simulink model "AariaHIABR2017a"  (R2017a)
settings: Solver=VariableStepAuto  StartTime=0.0  StopTime=inf  FixedStep=0.1  RelTol=1e-3  EnableMultiTasking=on
model workspace (MATLAB code in the model file):
  | my_a =1;
undefined symbols (not defined in the file or in its folder): AARIAENV, AARIAMAN, AARIASEN, Camera, sensor, Source_TS, X, Y, Z
libraries: sm_lib x347, nesl_utility x194, dspmathops x74, simulink x72, vrlib x2, powerlib_meascontrol x1, aerolibanimutils x1, aerolibutil x1
(part 1 of 9)
settings Model: Creator=mohmmadi  LastModifiedBy=hautakos
settings SolverCC: ZeroCrossControl=DisableAll  AutoInsertRateTranBlk=on
settings DataIOCC: LimitDataPoints=on  SaveOutput=off  SaveTime=off  ReturnWorkspaceOutputs=on
settings OptimizationCC: DefaultParameterBehavior=Inlined  InlineInvariantSignals=on  PassReuseOutputArgsThreshold=0  StateBitsets=on  DataBitsets=on  EfficientMapNaN2IntZero=off  LifeSpan=1
settings DebuggingCC: ReadBeforeWriteMsg=DisableAll  WriteAfterWriteMsg=DisableAll  WriteAfterReadMsg=DisableAll  MultiTaskDSMMsg=none  ParameterTunabilityLossMsg=error  AllowSymbolicDim=off  SFUnexpectedBacktrackingDiag=warning  SFNoUnconditionalDefaultTransitionDiag=warning  SFExecutionAtInitializationDiag=none
settings HardwareCC: ProdBitPerPointer=32  ProdBitPerSizeT=32  ProdBitPerPtrDiffT=32  ProdLargestAtomicFloat=None  ProdIntDivRoundTo=Floor  ProdWordSize=32  ProdHWDeviceType=Generic->Custom  TargetBitPerPointer=64  TargetBitPerSizeT=64  TargetBitPerPtrDiffT=64  TargetLongLongMode=on  TargetIntDivRoundTo=Zero  TargetEndianess=LittleEndian  TargetWordSize=64  TargetHWDeviceType=MATLAB Host  ProdEqTarget=off
settings ModelReferenceCC: UpdateModelReferenceTargets=IfOutOfDate  PropagateSignalLabelsOutOfModel=off
settings SFSimCC: SFSimEcho=off  MATLABDynamicMemAlloc=off
settings CodeAppCC: MaxIdLength=128
settings GRTTargetCC: TargetLangStandard=C89/C90 (ANSI)  CombineOutputUpdateFcns=off  GRTInterface=on
settings ConfigComp: CovMetricSettings=dw  CovHtmlReporting=on  CovSaveCumulativeToWorkspaceVar=on  CovSaveSingleToWorkspaceVar=on  CovExternalEMLEnable=off
settings ConfigurationSet: Description=SimMechanics 2G
settings ExplorerConfigSet: InternalSimMechanicsExplorerSettings="<ExplorerConfiguration><canonicalview>default</canonicalview><AnimationSetting><BasePlaybackSpeed>1.0</BasePlaybackSpeed><PlaybackSpeedFactor>2.0</PlaybackSpeedFactor></AnimationSetting><TilePanel><TileInfo><Tiles Columns=\"1\" Count=\"2\" Rows=\"2\"><Column Left=\"2\" Weight=\"1\"/><Column Left=\"662\"/><Row Top=\"2\" Weight=\"0.0567\"/><Row Top=\"65\" Weight=\"0.9433\"/><Row Top=\"1044\"/><Tile Height=\"1\" Width=\"1\" X=\"0\" Y=\"0\"/><Tile Height=\"1\" Width=\"1\" X=\"0\" Y=\"1\"/></Tiles></TileInfo><SceneInfo><SceneViewer><BGColor><R>0.60000002384185791</R><G>0.60000002384185791</G><B>0.60000002384185791</B></BGColor><Camera><DoPerspective>on</DoPerspective><Position><X>0.29999999999996857</X><Y>0.67968092512139899</Y><Z>1.3121696311764592</Z></Position><Center><X>-0.40710678118653471</X><Y>0.96126383425833517</Y><Z>1.9607920677927408</Z></Center><Up><X>-0.70710678118659176</X><Y>-0.28158290913685957</Y><Z>-0.64862243661621855</Z></Up><ViewLimDist>1</ViewLimDist><YLim>0.46630765815499858</YLim><XLim>5.6215978788685943</XLim></Camera></SceneViewer><SceneViewer><BGColor><R>0.60000002384185791</R><G>0.60000002384185791</G><B>0.60000002384185791</B></BGColor><Camera><DoPerspective>off</DoPerspective><Position><X>11.797763851673334</X><Y>-2.3957368450041248</Y><Z>7.7621866671693311</Z></Position><Center><X>-0.83316578837101418</X><Y>0.55050667633401429</Y><Z>1.2511357928731988</Z></Center><Up><X>-0.41467681338169138</X><Y>0.18924346197555764</Y><Z>0.89007306022770494</Z></Up><ViewLimDist>1</ViewLimDist><YLim>3.9492259066518822</YLim><XLim>2.6504598610622425</XLim></Camera></SceneViewer></SceneInfo></TilePanel><MechEditorPanel><Cameras><Camera><Id>Camera1</Id><Value><Name>Camera1</Name><NativeCamera><PositionTrackingFeature>Tool.Camera.R</PositionTrackingFeature><CenterTrackingFeature>Tool.Camera.R</CenterTrackingFeature><UpVectorTrackingFeature>Tool.Camera.R</UpVectorTrackingFeature><CenterTrackingOrigin>off</CenterTrackingOrigin><CenterTrackingDirection>+X</CenterTrackingDirection><UpVectorTrackingDirection>+Z</UpVectorTrackingDirection></NativeCamera></Value></Camera></Cameras><GfxPanelCameraMap><MapElement CameraMLId=\"Camera1\" GfxPanelIndex=\"0\"/></GfxPanelCameraMap><VideoCreator><PlaybackSpeedRatio>1.0</PlaybackSpeedRatio><FrameRate>30</FrameRate><VideoFormat>Motion JPEG AVI</VideoFormat><FrameSize>auto</FrameSize></VideoCreator></MechEditorPanel></ExplorerConfiguration>"

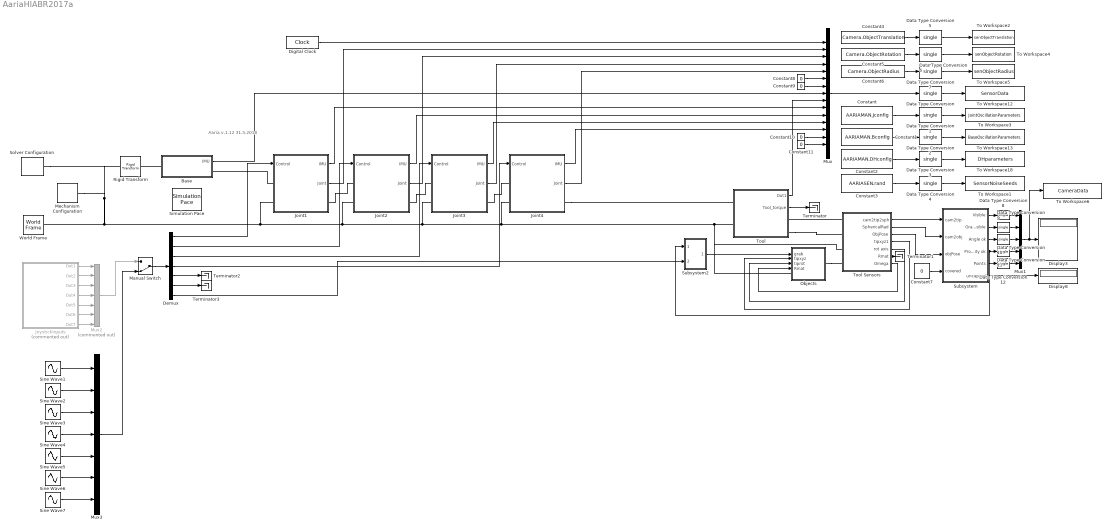
== system AariaHIABR2017a ==
  note: Aaria v.1.12
      | 31.5.2018
  Base : Subsystem  mask{Link_number=8}
  Constant : Constant  Value=AARIAMAN.Jconfig  VectorParams1D=off
  Constant1 : Constant  Value=AARIAMAN.Bconfig  VectorParams1D=off
  Constant{7..11} (5 alike) : Constant  Value=0
  Constant2 : Constant  Value=AARIAMAN.DHconfig  VectorParams1D=off  OutDataTypeStr=double
  Constant3 : Constant  Value=AARIASEN.rand  VectorParams1D=off  OutDataTypeStr=double
  Constant4 : Constant  Value=Camera.ObjectTranslation
  Constant5 : Constant  Value=Camera.ObjectRotation
  Constant6 : Constant  Value=Camera.ObjectRadius
  Data Type Conversion{,1..12} (13 alike) : DataTypeConversion  OutDataTypeStr=single
  Demux : Demux  Outputs=7
  Digital Clock : DigitalClock  SampleTime=AARIAENV.Sensor_TS
  Display3 : Display
  Display8 : Display
  Joint1 : Subsystem  mask{Link_number=1}
  Joint2 : Subsystem  mask{Link_number=2}
  Joint3 : Subsystem  mask{Link_number=3}
  Joint4 : Subsystem  mask{Link_number=4}
  JoystickInputs : Subsystem  Commented=on
  Manual Switch : ManualSwitch  CurrentSetting=0
  Mechanism Configuration : sm_lib/Utilities/Mechanism Configuration  UniformGravity=Constant  GravityVector=AARIAENV.gravity  GravityUnits=m/s^2  LinearizationDelta=0.001
  Mux : Mux  Inputs=15
  Mux1 : Mux  Inputs=5
  Mux2 : Mux  Commented=on  Inputs=7
  Mux3 : Mux  Inputs=7
  Objects : Subsystem
  Rigid Transform : sm_lib/Frames and Transforms/Rigid Transform  TranslationMethod=None  TranslationStandardOffset=0  TranslationLengthUnit=m  TranslationStandardAxis=+Z  TranslationCartesianOffset=[0 0 0.01]  TranslationROffset=0  TranslationROffsetUnits=m  TranslationZOffset=0  TranslationZOffsetUnits=m  TranslationThetaOffset=0  TranslationThetaOffsetUnits=deg  RotationMethod=StandardAxis  RotationAngleUnits=rad  RotationStandardAxis=+X  RotationAngle=-pi/2  RotationArbitraryAxis=[0 0 1]  FollAlignAxisA=+X  BaseAlignAxisA=+Y  FollAlignAxisB=+Y  BaseAlignAxisB=+Z  RotationSequenceAxes=FollowerAxes  RotationSequence=XYX  RotationSequenceAngles=[0 0 0]  RotationSequenceAnglesUnits=deg  RotationMatrix=[1 0 0; 0 1 0; 0 0 1]
  Simulation Pace : aerolibanimutils/Simulation Pace  SimulationPace=1  SleepMode=MATLAB Thread  OutputPaceError=off  SampleTime=1/30
  Sine Wave{1..7} (7 alike) : Sin  SampleTime=AARIAENV.Source_TS
  Solver Configuration : nesl_utility/Solver Configuration  PhysicalDomain=network_engine_domain  SubClassName=solver  LeftPortType=input  RightPortType=generic  Accelerate=off  Tones=[]  Harmonics=[]  SimulateNoise=off  Profile=off  UseLocalSampling=off  EnableSwitchedLinearOptims=on  FrequencyDomain=off  UseCCode=off  RelTol=0.001  AbsTol=1e-06  MinStep=1e-09  ToWorkspace=off  RevertToSquareIcSolve=off  NumHomotopyIterations=100  PhasorMode=off  PhasorModeNumHarmonics=1  OverrideAbsTol=off  DoDC=off  ResidualTolerance=1e-09  UseLocalSolver=off  LocalSolverChoice=NE_BACKWARD_EULER_ADVANCER  LocalSolverSampleTime=0.001  DoFixedCost=off  MaxNonlinIter=3  MaxModeIter=2  LinearAlgebra=Sparse  DelaysMemoryBudget=1024  AutomaticFiltering=on  FilteringTimeConstant=0.001
  Subsystem : Subsystem
  Subsystem2 : Subsystem
  Terminator{,1..3} (4 alike) : Terminator
  To Workspace1 : ToWorkspace  VariableName=SensorNoiseSeeds  SampleTime=AARIAENV.Sensor_TS
      settings: MaxDataPoints=8  Save2DSignal=2-D array (concatenate along first dimension)
  To Workspace12 : ToWorkspace  VariableName=SensorData  SampleTime=AARIAENV.Sensor_TS
      settings: Save2DSignal=2-D array (concatenate along first dimension)
  To Workspace13 : ToWorkspace  VariableName=BaseOscillationParameters  SampleTime=AARIAENV.Sensor_TS
      settings: MaxDataPoints=24  Save2DSignal=2-D array (concatenate along first dimension)
  To Workspace18 : ToWorkspace  VariableName=DHparameters  SampleTime=AARIAENV.Sensor_TS
      settings: MaxDataPoints=8  Save2DSignal=2-D array (concatenate along first dimension)
  To Workspace2 : ToWorkspace  VariableName=senObjectTranslation  SampleTime=AARIAENV.Sensor_TS
      settings: MaxDataPoints=1  Save2DSignal=2-D array (concatenate along first dimension)
  To Workspace3 : ToWorkspace  VariableName=JointOscillationParameters  SampleTime=AARIAENV.Sensor_TS
      settings: MaxDataPoints=6  Save2DSignal=2-D array (concatenate along first dimension)
  To Workspace4 : ToWorkspace  VariableName=senObjectRotation  SampleTime=AARIAENV.Sensor_TS
      settings: MaxDataPoints=3  Save2DSignal=2-D array (concatenate along first dimension)
  To Workspace5 : ToWorkspace  VariableName=senObjectRadius  SampleTime=AARIAENV.Sensor_TS
      settings: MaxDataPoints=1  Save2DSignal=2-D array (concatenate along first dimension)
  To Workspace6 : ToWorkspace  VariableName=CameraData  SampleTime=AARIAENV.Sensor_TS
      settings: Save2DSignal=2-D array (concatenate along first dimension)
  Tool : Subsystem  mask{Link_number=7}
  Tool Sensors : Subsystem
  World Frame : sm_lib/Frames and Transforms/World Frame
  wires:
  Data Type Conversion3/1 -> To Workspace18/1
  Constant2/1 -> Data Type Conversion3/1
  Data Type Conversion2/1 -> To Workspace13/1
  Joint3/2(Joint) -> Mux/4
  Joint1/2(Joint) -> Mux/2
  Data Type Conversion1/1 -> To Workspace3/1
  Data Type Conversion/1 -> To Workspace12/1
  Joint4/1(IMU) -> Mux/13
  Constant1/1 -> Data Type Conversion2/1
  Constant/1 -> Data Type Conversion1/1
  Tool/1(Out1) -> Mux/9
  Mux/1 -> Data Type Conversion/1
  Joint3/1(IMU) -> Mux/12
  Joint2/1(IMU) -> Mux/11
  Joint4/2(Joint) -> Mux/5
  Base/1(IMU) -> Mux/8
  Joint1/1(IMU) -> Mux/10
  Digital Clock/1 -> Mux/1
  Joint2/2(Joint) -> Mux/3
  Constant3/1 -> Data Type Conversion4/1
  Data Type Conversion4/1 -> To Workspace1/1
  Tool/2(Tool_torque) -> Terminator/1
  Data Type Conversion5/1 -> To Workspace2/1
  Constant5/1 -> Data Type Conversion6/1
  Constant6/1 -> Data Type Conversion7/1
  Data Type Conversion6/1 -> To Workspace4/1
  Constant4/1 -> Data Type Conversion5/1
  Data Type Conversion7/1 -> To Workspace5/1
  Tool Sensors/7(Omega) -> Objects/4(Rmat)
  Tool Sensors/3(ObjPose) -> Subsystem/3(objPose)
  Constant7/1 -> Subsystem/4(covered)
  Subsystem/1(Visible) -> Data Type Conversion8/1
  Subsystem/3(Angle ok) -> Data Type Conversion10/1
  Tool Sensors/6(Rmat) -> Terminator1/1
  Tool Sensors/1(cam2tip2sph) -> Subsystem/1(cam2tip)
  Subsystem/6(uncapped) -> Display8/1
  Tool Sensors/2(SphericalRad) -> Subsystem/2(cam2obj)
  Subsystem/5(Points) -> Data Type Conversion12/1
  Subsystem/2(Grab possible) -> Data Type Conversion9/1
  Mux1/1 -> To Workspace6/1, Display3/1
  Tool Sensors/5(rot axis) -> Objects/3(tiprot)
  Tool Sensors/4(tipxyz1) -> Objects/2(tipxyz)
  Demux/1 -> Joint1/1(Control)
  Demux/2 -> Joint2/1(Control)
  Demux/3 -> Joint3/1(Control)
  Demux/4 -> Joint4/1(Control)
  Data Type Conversion8/1 -> Mux1/1
  Data Type Conversion9/1 -> Mux1/2
  Data Type Conversion10/1 -> Mux1/3
  Data Type Conversion11/1 -> Mux1/4
  Data Type Conversion12/1 -> Mux1/5
  Demux/7 -> Subsystem2/2(GrabInput)
  Subsystem2/1(Out) -> Objects/1(grab)
  JoystickInputs/3(Out3) -> Mux2/3
  JoystickInputs/2(Out2) -> Mux2/2
  JoystickInputs/4(Out4) -> Mux2/4
  JoystickInputs/1(Out1) -> Mux2/1
  JoystickInputs/5(Out5) -> Mux2/5
  JoystickInputs/6(Out6) -> Mux2/6
  JoystickInputs/7(Out7) -> Mux2/7
  Sine Wave2/1 -> Mux3/2
  Sine Wave3/1 -> Mux3/3
  Sine Wave1/1 -> Mux3/1
  Sine Wave4/1 -> Mux3/4
  Sine Wave5/1 -> Mux3/5
  Sine Wave6/1 -> Mux3/6
  Sine Wave7/1 -> Mux3/7
  Manual Switch/1 -> Demux/1
  Mux2/1 -> Manual Switch/1
  Mux3/1 -> Manual Switch/2
  Constant8/1 -> Mux/6
  Constant9/1 -> Mux/7
  Constant10/1 -> Mux/14
  Constant11/1 -> Mux/15
  Demux/5 -> Terminator2/1
  Demux/6 -> Terminator3/1
  Subsystem/4(Proximity ok) -> Subsystem2/1(GrabPossible), Data Type Conversion11/1
  connections:
  Joint3/LConn1 -- Joint2/RConn1
  Tool/LConn2 -- Objects/LConn1 -- Tool Sensors/LConn3 -- Joint4/LConn2 -- Joint3/LConn2 -- Joint2/LConn2 -- Rigid Transform/LConn1 -- Solver Configuration/RConn1 -- Mechanism Configuration/RConn1 -- World Frame/RConn1 -- Joint1/LConn2
  Joint4/LConn1 -- Joint3/RConn1
  Joint4/RConn1 -- Tool/LConn1
  Joint2/LConn1 -- Joint1/RConn1
  Tool Sensors/LConn1 -- Tool/RConn1
  Tool/RConn2 -- Tool Sensors/LConn2
  Objects/RConn1 -- Tool Sensors/LConn4
  Joint1/LConn1 -- Base/RConn1
  Base/LConn1 -- Rigid Transform/RConn1

== system AariaHIABR2017a/Base ==
  BaseVSS : Subsystem  Variant=on  OverrideUsingVariant=VSS_MODE8 == 0  mask{Link_number=Link_number}
  Base : PMIOPort  Port=1  Side=Left
  Follower : PMIOPort  Port=2  Side=Right
  IMU : Outport
  wires:
  BaseVSS/1(IMU) -> IMU/1
  connections:
  Follower/RConn1 -- BaseVSS/RConn1
  Base/RConn1 -- BaseVSS/LConn1

== system AariaHIABR2017a/Joint1 ==
  note: Each join has to be configured in simulink after duplicating a module
      | Variant subsystem> block parameters > variant manager
      | Change the number the the end of Variant Control values to correspond
      | to the current joint. e.g Joint 3 variant control: VSS_MODE3 == ...
      | Conditions are automatically set to (N/A)
  Control : Inport
  RevoluteMotion : Subsystem  VariantControl=VSS_MODE1 == 1
  Base : PMIOPort  Port=1  Side=Left
  Follower : PMIOPort  Port=2  Side=Right
  Reference coord : PMIOPort  Port=3  Side=Left
  IMU : Outport
  Joint : Outport  Port=2
  wires:
  RevoluteMotion/1(IMU) -> IMU/1
  RevoluteMotion/2(Joint) -> Joint/1
  Control/1 -> RevoluteMotion/1(Control)
  connections:
  RevoluteMotion/RConn1 -- Follower/RConn1
  Base/RConn1 -- RevoluteMotion/LConn1
  Reference coord/RConn1 -- RevoluteMotion/LConn2

== system AariaHIABR2017a/Joint2 ==
  note: Each join has to be configured in simulink after duplicating a module
      | Variant subsystem> block parameters > variant manager
      | Change the number the the end of Variant Control values to correspond
      | to the current joint. e.g Joint 3 variant control: VSS_MODE3 == ...
      | Conditions are automatically set to (N/A)
  Control : Inport
  RevoluteMotion : Subsystem  VariantControl=VSS_MODE1 == 1
  Base : PMIOPort  Port=1  Side=Left
  Follower : PMIOPort  Port=2  Side=Right
  Reference coord : PMIOPort  Port=3  Side=Left
  IMU : Outport
  Joint : Outport  Port=2
  wires:
  Control/1 -> RevoluteMotion/1(Control)
  RevoluteMotion/2(Joint) -> Joint/1
  RevoluteMotion/1(IMU) -> IMU/1
  connections:
  Reference coord/RConn1 -- RevoluteMotion/LConn2
  Base/RConn1 -- RevoluteMotion/LConn1
  RevoluteMotion/RConn1 -- Follower/RConn1

== system AariaHIABR2017a/Joint3 ==
  note: Each join has to be configured in simulink after duplicating a module
      | Variant subsystem> block parameters > variant manager
      | Change the number the the end of Variant Control values to correspond
      | to the current joint. e.g Joint 3 variant control: VSS_MODE3 == ...
      | Conditions are automatically set to (N/A)
  Control : Inport
  RevoluteMotion : Subsystem  VariantControl=VSS_MODE1 == 1
  Base : PMIOPort  Port=1  Side=Left
  Follower : PMIOPort  Port=2  Side=Right
  Reference coord : PMIOPort  Port=3  Side=Left
  IMU : Outport
  Joint : Outport  Port=2
  wires:
  RevoluteMotion/1(IMU) -> IMU/1
  RevoluteMotion/2(Joint) -> Joint/1
  Control/1 -> RevoluteMotion/1(Control)
  connections:
  RevoluteMotion/RConn1 -- Follower/RConn1
  RevoluteMotion/LConn1 -- Base/RConn1
  Reference coord/RConn1 -- RevoluteMotion/LConn2

== system AariaHIABR2017a/Joint4 ==
  note: Each join has to be configured in simulink after duplicating a module
      | Variant subsystem> block parameters > variant manager
      | Change the number the the end of Variant Control values to correspond
      | to the current joint. e.g Joint 3 variant control: VSS_MODE3 == ...
      | Conditions are automatically set to (N/A)
  Control : Inport
  PrismaticMotion : Subsystem  VariantControl=VSS_MODE4 == 2
  Base : PMIOPort  Port=1  Side=Left
  Follower : PMIOPort  Port=2  Side=Right
  Reference coord : PMIOPort  Port=3  Side=Left
  IMU : Outport
  Joint : Outport  Port=2
  wires:
  Control/1 -> PrismaticMotion/1(Control)
  PrismaticMotion/2(Joint) -> Joint/1
  PrismaticMotion/1(IMU) -> IMU/1
  connections:
  Reference coord/RConn1 -- PrismaticMotion/LConn2
  Base/RConn1 -- PrismaticMotion/LConn1
  PrismaticMotion/RConn1 -- Follower/RConn1

== system AariaHIABR2017a/JoystickInputs ==
  Digital Clock1 : DigitalClock  SampleTime=AARIAENV.Sensor_TS
  Digital Clock2 : DigitalClock  Commented=on  SampleTime=AARIAENV.Sensor_TS
  Mux1 : Mux  Inputs=8
  Mux2 : Mux  Commented=on  Inputs=8
  Terminator{,1..6} (7 alike) : Terminator
  To Workspace : ToWorkspace  VariableName=JoystickData  SampleTime=-1
      settings: Save2DSignal=2-D array (concatenate along first dimension)
  To Workspace1 : ToWorkspace  Commented=on  VariableName=JoystickData2  SampleTime=-1
      settings: Save2DSignal=2-D array (concatenate along first dimension)
  Variant Subsystem : Subsystem  Variant=on
  Variant Subsystem1 : Subsystem  Commented=on  Variant=on
  Out1 : Outport
  Out2 : Outport  Port=2
  Out3 : Outport  Port=3
  Out4 : Outport  Port=4
  Out5 : Outport  Port=5
  Out6 : Outport  Port=6
  Out7 : Outport  Port=7
  wires:
  Variant Subsystem/2(Out2) -> Out2/1, Mux1/3
  Variant Subsystem/4(Out4) -> Mux1/5, Out4/1
  Variant Subsystem/3(Out3) -> Mux1/4, Out3/1
  Mux1/1 -> To Workspace/1
  Variant Subsystem/5(Out5) -> Mux1/6, Out5/1
  Variant Subsystem/6(Out6) -> Mux1/7, Out6/1
  Digital Clock1/1 -> Mux1/1
  Variant Subsystem/1(Out1) -> Out1/1, Mux1/2
  Variant Subsystem/7(Out7) -> Out7/1, Mux1/8
  Variant Subsystem1/7(Out7) -> Mux2/8, Terminator6/1
  Variant Subsystem1/1(Out1) -> Mux2/2, Terminator/1
  Digital Clock2/1 -> Mux2/1
  Variant Subsystem1/6(Out6) -> Mux2/7, Terminator5/1
  Variant Subsystem1/5(Out5) -> Mux2/6, Terminator4/1
  Mux2/1 -> To Workspace1/1
  Variant Subsystem1/3(Out3) -> Mux2/4, Terminator2/1
  Variant Subsystem1/4(Out4) -> Mux2/5, Terminator3/1
  Variant Subsystem1/2(Out2) -> Mux2/3, Terminator1/1

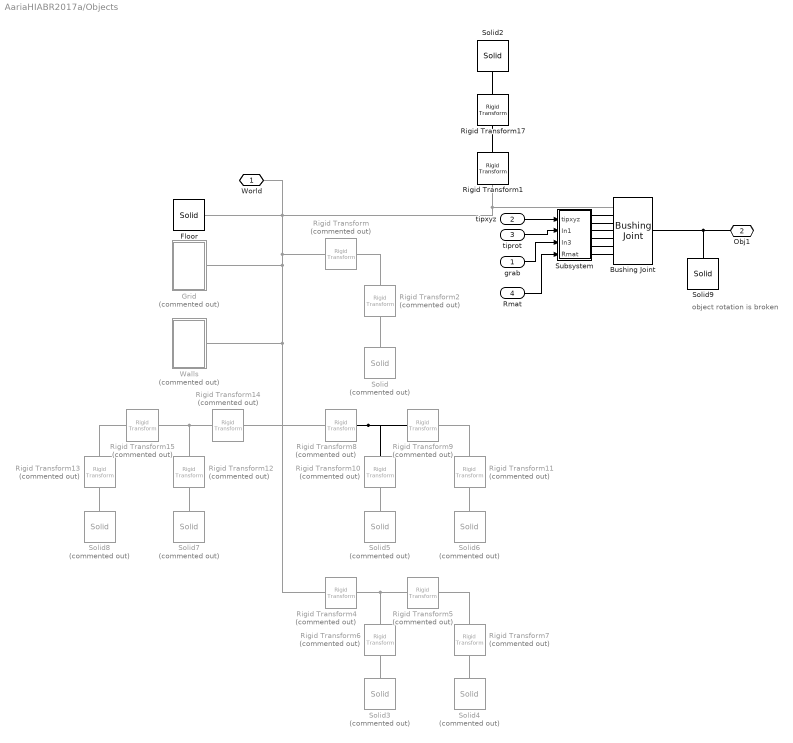
== system AariaHIABR2017a/Objects ==
  note: object rotation is broken
  grab : Inport
  tipxyz : Inport  Port=2
  tiprot : Inport  Port=3
  Rmat : Inport  Port=4
  Bushing Joint : sm_lib/Joints/Bushing Joint  SenseConstraintForce=off  SenseConstraintForceX=off  SenseConstraintForceY=off  SenseConstraintForceZ=off  SenseConstraintTorque=off  SenseConstraintTorqueX=off  SenseConstraintTorqueY=off  SenseConstraintTorqueZ=off  SenseTotalForce=off  SenseTotalForceX=off  SenseTotalForceY=off  SenseTotalForceZ=off  SenseTotalTorque=off  SenseTotalTorqueX=off  SenseTotalTorqueY=off  SenseTotalTorqueZ=off  CompositeWrenchDir=FollowerOnBase  CompositeWrenchFrame=BaseFrame  PxEquilibriumPosition=0  PxEquilibriumPositionUnits=m  PxSpringStiffness=0  PxSpringStiffnessUnits=N/m  PxDampingCoefficient=0  PxDampingCoefficientUnits=N/(m/s)  PxTorqueActuationMode=ComputedTorque  PxMotionActuationMode=InputMotion  PxSensePosition=off  PxSenseVelocity=off  PxSenseAcceleration=off  PxSenseTorqueForce=off  PxPositionTargetSpecify=off  PxPositionTargetPriority=High  PxPositionTargetValue=0  PxPositionTargetValueUnits=m  PxVelocityTargetSpecify=off  PxVelocityTargetPriority=High  PxVelocityTargetValue=0  PxVelocityTargetValueUnits=m/s  PyEquilibriumPosition=0  PyEquilibriumPositionUnits=m  PySpringStiffness=0  PySpringStiffnessUnits=N/m  PyDampingCoefficient=0  PyDampingCoefficientUnits=N/(m/s)  PyTorqueActuationMode=ComputedTorque  PyMotionActuationMode=InputMotion  PySensePosition=off  PySenseVelocity=off  PySenseAcceleration=off  PySenseTorqueForce=off  PyPositionTargetSpecify=off  PyPositionTargetPriority=High  PyPositionTargetValue=0  PyPositionTargetValueUnits=m  PyVelocityTargetSpecify=off  PyVelocityTargetPriority=High  PyVelocityTargetValue=0  PyVelocityTargetValueUnits=m/s  PzEquilibriumPosition=0  PzEquilibriumPositionUnits=m  PzSpringStiffness=0  PzSpringStiffnessUnits=N/m  PzDampingCoefficient=0  PzDampingCoefficientUnits=N/(m/s)  PzTorqueActuationMode=ComputedTorque  PzMotionActuationMode=InputMotion  PzSensePosition=off  PzSenseVelocity=off  PzSenseAcceleration=off  PzSenseTorqueForce=off  PzPositionTargetSpecify=off  PzPositionTargetPriority=High  PzPositionTargetValue=0  PzPositionTargetValueUnits=m  PzVelocityTargetSpecify=off  PzVelocityTargetPriority=High  PzVelocityTargetValue=0  PzVelocityTargetValueUnits=m/s  RxEquilibriumPosition=0  RxEquilibriumPositionUnits=deg  RxSpringStiffness=0  RxSpringStiffnessUnits=N*m/deg  RxDampingCoefficient=0  RxDampingCoefficientUnits=N*m/(deg/s)  RxTorqueActuationMode=ComputedTorque  RxMotionActuationMode=InputMotion  RxSensePosition=off  RxSenseVelocity=off  RxSenseAcceleration=off  RxSenseTorqueForce=off  RxPositionTargetSpecify=off  RxPositionTargetPriority=High  RxPositionTargetValue=pi/4  RxPositionTargetValueUnits=rad  RxVelocityTargetSpecify=off  RxVelocityTargetPriority=High  RxVelocityTargetValue=0  RxVelocityTargetValueUnits=deg/s  RyEquilibriumPosition=0  RyEquilibriumPositionUnits=deg  RySpringStiffness=0  RySpringStiffnessUnits=N*m/deg  RyDampingCoefficient=0  RyDampingCoefficientUnits=N*m/(deg/s)  RyTorqueActuationMode=ComputedTorque  RyMotionActuationMode=InputMotion  RySensePosition=off  RySenseVelocity=off  RySenseAcceleration=off  RySenseTorqueForce=off  RyPositionTargetSpecify=off  RyPositionTargetPriority=High  RyPositionTargetValue=0  RyPositionTargetValueUnits=deg  RyVelocityTargetSpecify=off  RyVelocityTargetPriority=High  RyVelocityTargetValue=0  RyVelocityTargetValueUnits=deg/s  RzEquilibriumPosition=0  RzEquilibriumPositionUnits=deg  RzSpringStiffness=0  RzSpringStiffnessUnits=N*m/deg  RzDampingCoefficient=0  RzDampingCoefficientUnits=N*m/(deg/s)  RzTorqueActuationMode=ComputedTorque  RzMotionActuationMode=InputMotion  RzSensePosition=off  RzSenseVelocity=off  RzSenseAcceleration=off  RzSenseTorqueForce=off  RzPositionTargetSpecify=off  RzPositionTargetPriority=High  RzPositionTargetValue=0  RzPositionTargetValueUnits=deg  RzVelocityTargetSpecify=off  RzVelocityTargetPriority=High  RzVelocityTargetValue=0  RzVelocityTargetValueUnits=deg/s
      settings: SourceProductName=Simscape Multibody
  Floor : sm_lib/Body Elements/Solid  InertiaType=CalculateFromGeometry  Mass=1  MassUnits=kg  CenterOfMass=[0 0 0]  CenterOfMassUnits=m  MomentsOfInertia=[1 1 1]  MomentsOfInertiaUnits=kg*m^2  ProductsOfInertia=[1 1 1]  ProductsOfInertiaUnits=kg*m^2  DensityBased=on  Density=1000  DensityUnits=kg/m^3  DoExposeReferenceFrame=on  SerializedFrames=<Frames/>  GraphicType=FromGeometry  MarkerShape=Sphere  MarkerSize=10  GraphicVisPropType=SimpleVisualProperties  GraphicDiffuseColor=[0.5 0.5 0.5]  GraphicSpecularColor=[0.5 0.5 0.5 1.0]  GraphicAmbientColor=[0.15 0.15 0.15 1.0]  GraphicEmissiveColor=[0.0 0.0 0.0 1.0]  GraphicShininess=75  GraphicOpacity=1.0  GeometryShape=Brick  RectangleSize=[1 1]  RectangleSizeUnits=m  BrickDimensions=[20 20 0.1]  BrickDimensionUnits=m  CylinderRadius=1  CylinderRadiusUnits=m  CylinderLength=1  CylinderLengthUnits=m  SphereRadius=1  SphereRadiusUnits=m  EllipsoidRadii=[1 1 1]  EllipsoidRadiiUnits=m  ExtrusionCrossSection=[1 1; -1 1; -1 -1; 1 -1]  ExtrusionCrossSectionUnits=m  ExtrusionLength=1  ExtrusionLengthUnits=m  PolygonNumSides=3  PolygonOuterRadius=1  PolygonOuterRadiusUnits=m  ExtGeomFileType=STEP  ExtGeomFileUnits=m  RevolutionCrossSection=[1 1; 1 -1; 2 -1; 2 1]  RevolutionCrossSectionUnits=m  RevolutionExtent=Full  RevolutionAngle=180  RevolutionAngleUnits=deg
  Grid : Subsystem  Commented=on
  Rigid Transform : sm_lib/Frames and Transforms/Rigid Transform  Commented=on  TranslationMethod=StandardAxis  TranslationStandardOffset=5  TranslationLengthUnit=m  TranslationStandardAxis=+Y  TranslationCartesianOffset=[0 0 0]  TranslationROffset=0  TranslationROffsetUnits=m  TranslationZOffset=0  TranslationZOffsetUnits=m  TranslationThetaOffset=0  TranslationThetaOffsetUnits=deg  RotationMethod=None  RotationAngleUnits=deg  RotationStandardAxis=+Z  RotationAngle=0.0  RotationArbitraryAxis=[0 0 1]  FollAlignAxisA=+X  BaseAlignAxisA=+Y  FollAlignAxisB=+Y  BaseAlignAxisB=+Z  RotationSequenceAxes=FollowerAxes  RotationSequence=XYX  RotationSequenceAngles=[0 0 0]  RotationSequenceAnglesUnits=deg  RotationMatrix=[1 0 0; 0 1 0; 0 0 1]
  Rigid Transform1 : sm_lib/Frames and Transforms/Rigid Transform  TranslationMethod=Cartesian  TranslationStandardOffset=4  TranslationLengthUnit=m  TranslationStandardAxis=+Y  TranslationCartesianOffset=Camera.ObjectTranslation  TranslationROffset=0  TranslationROffsetUnits=m  TranslationZOffset=0  TranslationZOffsetUnits=m  TranslationThetaOffset=0  TranslationThetaOffsetUnits=deg  RotationMethod=None  RotationAngleUnits=deg  RotationStandardAxis=+Z  RotationAngle=0.0  RotationArbitraryAxis=[0 0 1]  FollAlignAxisA=+X  BaseAlignAxisA=+Y  FollAlignAxisB=+Y  BaseAlignAxisB=+Z  RotationSequenceAxes=FollowerAxes  RotationSequence=XYX  RotationSequenceAngles=[0 0 0]  RotationSequenceAnglesUnits=deg  RotationMatrix=[1 0 0; 0 1 0; 0 0 1]
  Rigid Transform{2,6,10,12} (4 alike) : sm_lib/Frames and Transforms/Rigid Transform  Commented=on  TranslationMethod=StandardAxis  TranslationStandardOffset=0.25  TranslationLengthUnit=m  TranslationStandardAxis=+Z  TranslationCartesianOffset=[0 0 0]  TranslationROffset=0  TranslationROffsetUnits=m  TranslationZOffset=0  TranslationZOffsetUnits=m  TranslationThetaOffset=0  TranslationThetaOffsetUnits=deg  RotationMethod=StandardAxis  RotationAngleUnits=deg  RotationStandardAxis=+Z  RotationAngle=45  RotationArbitraryAxis=[0 0 1]  FollAlignAxisA=+X  BaseAlignAxisA=+Y  FollAlignAxisB=+Y  BaseAlignAxisB=+Z  RotationSequenceAxes=FollowerAxes  RotationSequence=XYX  RotationSequenceAngles=[0 0 0]  RotationSequenceAnglesUnits=deg  RotationMatrix=[1 0 0; 0 1 0; 0 0 1]
  Rigid Transform11 : sm_lib/Frames and Transforms/Rigid Transform  Commented=on  TranslationMethod=StandardAxis  TranslationStandardOffset=0.5  TranslationLengthUnit=m  TranslationStandardAxis=+Z  TranslationCartesianOffset=[0 0 0]  TranslationROffset=0  TranslationROffsetUnits=m  TranslationZOffset=0  TranslationZOffsetUnits=m  TranslationThetaOffset=0  TranslationThetaOffsetUnits=deg  RotationMethod=StandardAxis  RotationAngleUnits=deg  RotationStandardAxis=+Z  RotationAngle=30  RotationArbitraryAxis=[0 0 1]  FollAlignAxisA=+X  BaseAlignAxisA=+Y  FollAlignAxisB=+Y  BaseAlignAxisB=+Z  RotationSequenceAxes=FollowerAxes  RotationSequence=XYX  RotationSequenceAngles=[0 0 0]  RotationSequenceAnglesUnits=deg  RotationMatrix=[1 0 0; 0 1 0; 0 0 1]
  Rigid Transform13 : sm_lib/Frames and Transforms/Rigid Transform  Commented=on  TranslationMethod=StandardAxis  TranslationStandardOffset=0.5  TranslationLengthUnit=m  TranslationStandardAxis=+Z  TranslationCartesianOffset=[0 0 0]  TranslationROffset=0  TranslationROffsetUnits=m  TranslationZOffset=0  TranslationZOffsetUnits=m  TranslationThetaOffset=0  TranslationThetaOffsetUnits=deg  RotationMethod=StandardAxis  RotationAngleUnits=deg  RotationStandardAxis=+Z  RotationAngle=30  RotationArbitraryAxis=[0 0 1]  FollAlignAxisA=+X  BaseAlignAxisA=+Y  FollAlignAxisB=+Y  BaseAlignAxisB=+Z  RotationSequenceAxes=FollowerAxes  RotationSequence=XYX  RotationSequenceAngles=[0 0 0]  RotationSequenceAnglesUnits=deg  RotationMatrix=[1 0 0; 0 1 0; 0 0 1]
  Rigid Transform14 : sm_lib/Frames and Transforms/Rigid Transform  Commented=on  TranslationMethod=StandardAxis  TranslationStandardOffset=5  TranslationLengthUnit=m  TranslationStandardAxis=-X  TranslationCartesianOffset=[0 0 0]  TranslationROffset=0  TranslationROffsetUnits=m  TranslationZOffset=0  TranslationZOffsetUnits=m  TranslationThetaOffset=0  TranslationThetaOffsetUnits=deg  RotationMethod=None  RotationAngleUnits=deg  RotationStandardAxis=+Z  RotationAngle=0.0  RotationArbitraryAxis=[0 0 1]  FollAlignAxisA=+X  BaseAlignAxisA=+Y  FollAlignAxisB=+Y  BaseAlignAxisB=+Z  RotationSequenceAxes=FollowerAxes  RotationSequence=XYX  RotationSequenceAngles=[0 0 0]  RotationSequenceAnglesUnits=deg  RotationMatrix=[1 0 0; 0 1 0; 0 0 1]
  Rigid Transform15 : sm_lib/Frames and Transforms/Rigid Transform  Commented=on  TranslationMethod=StandardAxis  TranslationStandardOffset=1  TranslationLengthUnit=m  TranslationStandardAxis=-X  TranslationCartesianOffset=[0 0 0]  TranslationROffset=0  TranslationROffsetUnits=m  TranslationZOffset=0  TranslationZOffsetUnits=m  TranslationThetaOffset=0  TranslationThetaOffsetUnits=deg  RotationMethod=None  RotationAngleUnits=deg  RotationStandardAxis=+Z  RotationAngle=0.0  RotationArbitraryAxis=[0 0 1]  FollAlignAxisA=+X  BaseAlignAxisA=+Y  FollAlignAxisB=+Y  BaseAlignAxisB=+Z  RotationSequenceAxes=FollowerAxes  RotationSequence=XYX  RotationSequenceAngles=[0 0 0]  RotationSequenceAnglesUnits=deg  RotationMatrix=[1 0 0; 0 1 0; 0 0 1]
  Rigid Transform17 : sm_lib/Frames and Transforms/Rigid Transform  TranslationMethod=Cartesian  TranslationStandardOffset=0.5  TranslationLengthUnit=m  TranslationStandardAxis=+Z  TranslationCartesianOffset=[0 0 -Camera.ObjectTranslation(3)/2 ]  TranslationROffset=0  TranslationROffsetUnits=m  TranslationZOffset=0  TranslationZOffsetUnits=m  TranslationThetaOffset=0  TranslationThetaOffsetUnits=deg  RotationMethod=None  RotationAngleUnits=deg  RotationStandardAxis=+Z  RotationAngle=45  RotationArbitraryAxis=[0.4 0.9 1]  FollAlignAxisA=+X  BaseAlignAxisA=+Y  FollAlignAxisB=+Y  BaseAlignAxisB=+Z  RotationSequenceAxes=FollowerAxes  RotationSequence=XYX  RotationSequenceAngles=[0 0 0]  RotationSequenceAnglesUnits=deg  RotationMatrix=Camera.ObjectRotation
  Rigid Transform4 : sm_lib/Frames and Transforms/Rigid Transform  Commented=on  TranslationMethod=StandardAxis  TranslationStandardOffset=3  TranslationLengthUnit=m  TranslationStandardAxis=-Y  TranslationCartesianOffset=[0 0 0]  TranslationROffset=0  TranslationROffsetUnits=m  TranslationZOffset=0  TranslationZOffsetUnits=m  TranslationThetaOffset=0  TranslationThetaOffsetUnits=deg  RotationMethod=None  RotationAngleUnits=deg  RotationStandardAxis=+Z  RotationAngle=0.0  RotationArbitraryAxis=[0 0 1]  FollAlignAxisA=+X  BaseAlignAxisA=+Y  FollAlignAxisB=+Y  BaseAlignAxisB=+Z  RotationSequenceAxes=FollowerAxes  RotationSequence=XYX  RotationSequenceAngles=[0 0 0]  RotationSequenceAnglesUnits=deg  RotationMatrix=[1 0 0; 0 1 0; 0 0 1]
  Rigid Transform5 : sm_lib/Frames and Transforms/Rigid Transform  Commented=on  TranslationMethod=StandardAxis  TranslationStandardOffset=3  TranslationLengthUnit=m  TranslationStandardAxis=-Y  TranslationCartesianOffset=[0 0 0]  TranslationROffset=0  TranslationROffsetUnits=m  TranslationZOffset=0  TranslationZOffsetUnits=m  TranslationThetaOffset=0  TranslationThetaOffsetUnits=deg  RotationMethod=None  RotationAngleUnits=deg  RotationStandardAxis=+Z  RotationAngle=0.0  RotationArbitraryAxis=[0 0 1]  FollAlignAxisA=+X  BaseAlignAxisA=+Y  FollAlignAxisB=+Y  BaseAlignAxisB=+Z  RotationSequenceAxes=FollowerAxes  RotationSequence=XYX  RotationSequenceAngles=[0 0 0]  RotationSequenceAnglesUnits=deg  RotationMatrix=[1 0 0; 0 1 0; 0 0 1]
  Rigid Transform7 : sm_lib/Frames and Transforms/Rigid Transform  Commented=on  TranslationMethod=StandardAxis  TranslationStandardOffset=0.5  TranslationLengthUnit=m  TranslationStandardAxis=+Z  TranslationCartesianOffset=[0 0 0]  TranslationROffset=0  TranslationROffsetUnits=m  TranslationZOffset=0  TranslationZOffsetUnits=m  TranslationThetaOffset=0  TranslationThetaOffsetUnits=deg  RotationMethod=StandardAxis  RotationAngleUnits=deg  RotationStandardAxis=+Z  RotationAngle=30  RotationArbitraryAxis=[0 0 1]  FollAlignAxisA=+X  BaseAlignAxisA=+Y  FollAlignAxisB=+Y  BaseAlignAxisB=+Z  RotationSequenceAxes=FollowerAxes  RotationSequence=XYX  RotationSequenceAngles=[0 0 0]  RotationSequenceAnglesUnits=deg  RotationMatrix=[1 0 0; 0 1 0; 0 0 1]
  Rigid Transform8 : sm_lib/Frames and Transforms/Rigid Transform  Commented=on  TranslationMethod=StandardAxis  TranslationStandardOffset=5  TranslationLengthUnit=m  TranslationStandardAxis=+X  TranslationCartesianOffset=[0 0 0]  TranslationROffset=0  TranslationROffsetUnits=m  TranslationZOffset=0  TranslationZOffsetUnits=m  TranslationThetaOffset=0  TranslationThetaOffsetUnits=deg  RotationMethod=None  RotationAngleUnits=deg  RotationStandardAxis=+Z  RotationAngle=0.0  RotationArbitraryAxis=[0 0 1]  FollAlignAxisA=+X  BaseAlignAxisA=+Y  FollAlignAxisB=+Y  BaseAlignAxisB=+Z  RotationSequenceAxes=FollowerAxes  RotationSequence=XYX  RotationSequenceAngles=[0 0 0]  RotationSequenceAnglesUnits=deg  RotationMatrix=[1 0 0; 0 1 0; 0 0 1]
  Rigid Transform9 : sm_lib/Frames and Transforms/Rigid Transform  Commented=on  TranslationMethod=StandardAxis  TranslationStandardOffset=2  TranslationLengthUnit=m  TranslationStandardAxis=+X  TranslationCartesianOffset=[0 0 0]  TranslationROffset=0  TranslationROffsetUnits=m  TranslationZOffset=0  TranslationZOffsetUnits=m  TranslationThetaOffset=0  TranslationThetaOffsetUnits=deg  RotationMethod=None  RotationAngleUnits=deg  RotationStandardAxis=+Z  RotationAngle=0.0  RotationArbitraryAxis=[0 0 1]  FollAlignAxisA=+X  BaseAlignAxisA=+Y  FollAlignAxisB=+Y  BaseAlignAxisB=+Z  RotationSequenceAxes=FollowerAxes  RotationSequence=XYX  RotationSequenceAngles=[0 0 0]  RotationSequenceAnglesUnits=deg  RotationMatrix=[1 0 0; 0 1 0; 0 0 1]
  Solid{,3,5,7} (4 alike) : sm_lib/Body Elements/Solid  Commented=on  InertiaType=CalculateFromGeometry  Mass=1  MassUnits=kg  CenterOfMass=[0 0 0]  CenterOfMassUnits=m  MomentsOfInertia=[1 1 1]  MomentsOfInertiaUnits=kg*m^2  ProductsOfInertia=[1 1 1]  ProductsOfInertiaUnits=kg*m^2  DensityBased=on  Density=1000  DensityUnits=kg/m^3  DoExposeReferenceFrame=on  SerializedFrames=<Frames/>  GraphicType=FromGeometry  MarkerShape=Sphere  MarkerSize=10  GraphicVisPropType=SimpleVisualProperties  GraphicDiffuseColor=[0.0 0.0 1.0]  GraphicSpecularColor=[0.5 0.5 0.5 1.0]  GraphicAmbientColor=[0.15 0.15 0.15 1.0]  GraphicEmissiveColor=[0.0 0.0 0.0 1.0]  GraphicShininess=75  GraphicOpacity=1.0  GeometryShape=Brick  RectangleSize=[1 1]  RectangleSizeUnits=m  BrickDimensions=[0.5 0.5 0.5]  BrickDimensionUnits=m  CylinderRadius=1  CylinderRadiusUnits=m  CylinderLength=1  CylinderLengthUnits=m  SphereRadius=1  SphereRadiusUnits=m  EllipsoidRadii=[1 1 1]  EllipsoidRadiiUnits=m  ExtrusionCrossSection=[1 1; -1 1; -1 -1; 1 -1]  ExtrusionCrossSectionUnits=m  ExtrusionLength=1  ExtrusionLengthUnits=m  PolygonNumSides=3  PolygonOuterRadius=1  PolygonOuterRadiusUnits=m  ExtGeomFileType=STEP  ExtGeomFileUnits=m  RevolutionCrossSection=[1 1; 1 -1; 2 -1; 2 1]  RevolutionCrossSectionUnits=m  RevolutionExtent=Full  RevolutionAngle=180  RevolutionAngleUnits=deg
  Solid2 : sm_lib/Body Elements/Solid  InertiaType=CalculateFromGeometry  Mass=1  MassUnits=kg  CenterOfMass=[0 0 0]  CenterOfMassUnits=m  MomentsOfInertia=[1 1 1]  MomentsOfInertiaUnits=kg*m^2  ProductsOfInertia=[1 1 1]  ProductsOfInertiaUnits=kg*m^2  DensityBased=off  Density=1000  DensityUnits=kg/m^3  DoExposeReferenceFrame=on  SerializedFrames=<Frames/>  GraphicType=FromGeometry  MarkerShape=Sphere  MarkerSize=10  GraphicVisPropType=SimpleVisualProperties  GraphicDiffuseColor=[1.0 0.2 0.2]  GraphicSpecularColor=[0.5 0.5 0.5 1.0]  GraphicAmbientColor=[0.15 0.15 0.15 1.0]  GraphicEmissiveColor=[0.0 0.0 0.0 1.0]  GraphicShininess=75  GraphicOpacity=1.0  GeometryShape=Brick  RectangleSize=[1 1]  RectangleSizeUnits=m  BrickDimensions=[0.02 0.02 abs(Camera.ObjectTranslation(3))]  BrickDimensionUnits=m  CylinderRadius=1  CylinderRadiusUnits=m  CylinderLength=1  CylinderLengthUnits=m  SphereRadius=1  SphereRadiusUnits=m  EllipsoidRadii=[1 1 1]  EllipsoidRadiiUnits=m  ExtrusionCrossSection=[1 1; -1 1; -1 -1; 1 -1]  ExtrusionCrossSectionUnits=m  ExtrusionLength=1  ExtrusionLengthUnits=m  PolygonNumSides=3  PolygonOuterRadius=1  PolygonOuterRadiusUnits=m  ExtGeomFileType=STEP  ExtGeomFileUnits=m  RevolutionCrossSection=[1 1; 1 -1; 2 -1; 2 1]  RevolutionCrossSectionUnits=m  RevolutionExtent=Full  RevolutionAngle=180  RevolutionAngleUnits=deg
  Solid4 : sm_lib/Body Elements/Solid  Commented=on  InertiaType=CalculateFromGeometry  Mass=1  MassUnits=kg  CenterOfMass=[0 0 0]  CenterOfMassUnits=m  MomentsOfInertia=[1 1 1]  MomentsOfInertiaUnits=kg*m^2  ProductsOfInertia=[1 1 1]  ProductsOfInertiaUnits=kg*m^2  DensityBased=on  Density=1000  DensityUnits=kg/m^3  DoExposeReferenceFrame=on  SerializedFrames=<Frames/>  GraphicType=FromGeometry  MarkerShape=Sphere  MarkerSize=10  GraphicVisPropType=SimpleVisualProperties  GraphicDiffuseColor=[1.0 0.2 0.2]  GraphicSpecularColor=[0.5 0.5 0.5 1.0]  GraphicAmbientColor=[0.15 0.15 0.15 1.0]  GraphicEmissiveColor=[0.0 0.0 0.0 1.0]  GraphicShininess=75  GraphicOpacity=1.0  GeometryShape=Brick  RectangleSize=[1 1]  RectangleSizeUnits=m  BrickDimensions=[1 1 1]  BrickDimensionUnits=m  CylinderRadius=1  CylinderRadiusUnits=m  CylinderLength=1  CylinderLengthUnits=m  SphereRadius=1  SphereRadiusUnits=m  EllipsoidRadii=[1 1 1]  EllipsoidRadiiUnits=m  ExtrusionCrossSection=[1 1; -1 1; -1 -1; 1 -1]  ExtrusionCrossSectionUnits=m  ExtrusionLength=1  ExtrusionLengthUnits=m  PolygonNumSides=3  PolygonOuterRadius=1  PolygonOuterRadiusUnits=m  ExtGeomFileType=STEP  ExtGeomFileUnits=m  RevolutionCrossSection=[1 1; 1 -1; 2 -1; 2 1]  RevolutionCrossSectionUnits=m  RevolutionExtent=Full  RevolutionAngle=180  RevolutionAngleUnits=deg
  Solid6 : sm_lib/Body Elements/Solid  Commented=on  InertiaType=CalculateFromGeometry  Mass=1  MassUnits=kg  CenterOfMass=[0 0 0]  CenterOfMassUnits=m  MomentsOfInertia=[1 1 1]  MomentsOfInertiaUnits=kg*m^2  ProductsOfInertia=[1 1 1]  ProductsOfInertiaUnits=kg*m^2  DensityBased=on  Density=1000  DensityUnits=kg/m^3  DoExposeReferenceFrame=on  SerializedFrames=<Frames/>  GraphicType=FromGeometry  MarkerShape=Sphere  MarkerSize=10  GraphicVisPropType=SimpleVisualProperties  GraphicDiffuseColor=[1.0 0.2 0.2]  GraphicSpecularColor=[0.5 0.5 0.5 1.0]  GraphicAmbientColor=[0.15 0.15 0.15 1.0]  GraphicEmissiveColor=[0.0 0.0 0.0 1.0]  GraphicShininess=75  GraphicOpacity=1.0  GeometryShape=Brick  RectangleSize=[1 1]  RectangleSizeUnits=m  BrickDimensions=[1 1 1]  BrickDimensionUnits=m  CylinderRadius=1  CylinderRadiusUnits=m  CylinderLength=1  CylinderLengthUnits=m  SphereRadius=1  SphereRadiusUnits=m  EllipsoidRadii=[1 1 1]  EllipsoidRadiiUnits=m  ExtrusionCrossSection=[1 1; -1 1; -1 -1; 1 -1]  ExtrusionCrossSectionUnits=m  ExtrusionLength=1  ExtrusionLengthUnits=m  PolygonNumSides=3  PolygonOuterRadius=1  PolygonOuterRadiusUnits=m  ExtGeomFileType=STEP  ExtGeomFileUnits=m  RevolutionCrossSection=[1 1; 1 -1; 2 -1; 2 1]  RevolutionCrossSectionUnits=m  RevolutionExtent=Full  RevolutionAngle=180  RevolutionAngleUnits=deg
  Solid8 : sm_lib/Body Elements/Solid  Commented=on  InertiaType=CalculateFromGeometry  Mass=1  MassUnits=kg  CenterOfMass=[0 0 0]  CenterOfMassUnits=m  MomentsOfInertia=[1 1 1]  MomentsOfInertiaUnits=kg*m^2  ProductsOfInertia=[1 1 1]  ProductsOfInertiaUnits=kg*m^2  DensityBased=on  Density=1000  DensityUnits=kg/m^3  DoExposeReferenceFrame=on  SerializedFrames=<Frames/>  GraphicType=FromGeometry  MarkerShape=Sphere  MarkerSize=10  GraphicVisPropType=SimpleVisualProperties  GraphicDiffuseColor=[1.0 0.2 0.2]  GraphicSpecularColor=[0.5 0.5 0.5 1.0]  GraphicAmbientColor=[0.15 0.15 0.15 1.0]  GraphicEmissiveColor=[0.0 0.0 0.0 1.0]  GraphicShininess=75  GraphicOpacity=1.0  GeometryShape=Brick  RectangleSize=[1 1]  RectangleSizeUnits=m  BrickDimensions=[1 1 1]  BrickDimensionUnits=m  CylinderRadius=1  CylinderRadiusUnits=m  CylinderLength=1  CylinderLengthUnits=m  SphereRadius=1  SphereRadiusUnits=m  EllipsoidRadii=[1 1 1]  EllipsoidRadiiUnits=m  ExtrusionCrossSection=[1 1; -1 1; -1 -1; 1 -1]  ExtrusionCrossSectionUnits=m  ExtrusionLength=1  ExtrusionLengthUnits=m  PolygonNumSides=3  PolygonOuterRadius=1  PolygonOuterRadiusUnits=m  ExtGeomFileType=STEP  ExtGeomFileUnits=m  RevolutionCrossSection=[1 1; 1 -1; 2 -1; 2 1]  RevolutionCrossSectionUnits=m  RevolutionExtent=Full  RevolutionAngle=180  RevolutionAngleUnits=deg
  Solid9 : sm_lib/Body Elements/Solid  InertiaType=CalculateFromGeometry  Mass=1  MassUnits=kg  CenterOfMass=[0 0 0]  CenterOfMassUnits=m  MomentsOfInertia=[1 1 1]  MomentsOfInertiaUnits=kg*m^2  ProductsOfInertia=[1 1 1]  ProductsOfInertiaUnits=kg*m^2  DensityBased=on  Density=1000  DensityUnits=kg/m^3  DoExposeReferenceFrame=on  SerializedFrames=<Frames/>  GraphicType=FromGeometry  MarkerShape=Sphere  MarkerSize=10  GraphicVisPropType=SimpleVisualProperties  GraphicDiffuseColor=[1.0 1.0 0.0]  GraphicSpecularColor=[0.5 0.5 0.5 1.0]  GraphicAmbientColor=[0.15 0.15 0.15 1.0]  GraphicEmissiveColor=[0.0 0.0 0.0 1.0]  GraphicShininess=75  GraphicOpacity=1.0  GeometryShape=Brick  RectangleSize=[1 1]  RectangleSizeUnits=m  BrickDimensions=[Camera.ObjectRadius*2 Camera.ObjectRadius*2 Camera.ObjectRadius*2]  BrickDimensionUnits=m  CylinderRadius=1  CylinderRadiusUnits=m  CylinderLength=1  CylinderLengthUnits=m  SphereRadius=1  SphereRadiusUnits=m  EllipsoidRadii=[1 1 1]  EllipsoidRadiiUnits=m  ExtrusionCrossSection=[1 1; -1 1; -1 -1; 1 -1]  ExtrusionCrossSectionUnits=m  ExtrusionLength=1  ExtrusionLengthUnits=m  PolygonNumSides=3  PolygonOuterRadius=1  PolygonOuterRadiusUnits=m  ExtGeomFileType=STEP  ExtGeomFileUnits=m  RevolutionCrossSection=[1 1; 1 -1; 2 -1; 2 1]  RevolutionCrossSectionUnits=m  RevolutionExtent=Full  RevolutionAngle=180  RevolutionAngleUnits=deg
  Subsystem : Subsystem
  Walls : Subsystem  Commented=on
  World : PMIOPort  Port=1  Side=Left
  Obj1 : PMIOPort  Port=2  Side=Right
  wires:
  grab/1 -> Subsystem/3(In3)
  tipxyz/1 -> Subsystem/1(tipxyz)
  tiprot/1 -> Subsystem/2(In1)
  Rmat/1 -> Subsystem/4(Rmat)
  connections:
  Rigid Transform12/LConn1 -- Rigid Transform15/LConn1 -- Rigid Transform14/RConn1
  Rigid Transform8/RConn1 -- Rigid Transform9/LConn1 -- Rigid Transform10/LConn1
  Rigid Transform11/LConn1 -- Rigid Transform9/RConn1
  Solid7/RConn1 -- Rigid Transform12/RConn1
  Solid4/RConn1 -- Rigid Transform7/RConn1
  Rigid Transform2/LConn1 -- Rigid Transform/RConn1
  Solid3/RConn1 -- Rigid Transform6/RConn1
  Solid5/RConn1 -- Rigid Transform10/RConn1
  Solid8/RConn1 -- Rigid Transform13/RConn1
  Rigid Transform13/LConn1 -- Rigid Transform15/RConn1
  Rigid Transform7/LConn1 -- Rigid Transform5/RConn1
  Solid6/RConn1 -- Rigid Transform11/RConn1
  Rigid Transform6/LConn1 -- Rigid Transform5/LConn1 -- Rigid Transform4/RConn1
  Solid/RConn1 -- Rigid Transform2/RConn1
  Solid2/RConn1 -- Rigid Transform17/RConn1
  Subsystem/RConn1 -- Bushing Joint/LConn2
  Bushing Joint/LConn3 -- Subsystem/RConn2
  Bushing Joint/LConn4 -- Subsystem/RConn3
  Bushing Joint/LConn5 -- Subsystem/RConn4
  Bushing Joint/LConn6 -- Subsystem/RConn5
  Bushing Joint/LConn7 -- Subsystem/RConn6
  Rigid Transform/LConn1 -- Walls/LConn1 -- Rigid Transform14/LConn1 -- Rigid Transform4/LConn1 -- Rigid Transform8/LConn1 -- Grid/RConn1 -- Rigid Transform1/LConn1 -- Bushing Joint/LConn1 -- World/RConn1 -- Floor/RConn1
  Bushing Joint/RConn1 -- Solid9/RConn1 -- Obj1/RConn1
  Rigid Transform17/LConn1 -- Rigid Transform1/RConn1

== system AariaHIABR2017a/Subsystem ==
  cam2tip : Inport
  cam2obj : Inport  Port=2
  objPose : Inport  Port=3
  covered : Inport  Port=4
  FoV : Subsystem
  Mux : Mux
  Score : Subsystem
  grab_check_cam above angled down : Subsystem
  Visible : Outport
  Grab possible : Outport  Port=2
  Angle ok : Outport  Port=3
  Proximity ok : Outport  Port=4
  Points : Outport  Port=5
  uncapped : Outport  Port=6
  wires:
  grab_check_cam above angled down/3(orientation ok) -> Mux/4, Proximity ok/1
  grab_check_cam above angled down/2(pose ok) -> Mux/3, Angle ok/1
  covered/1 -> FoV/2(Covered)
  cam2tip/1 -> grab_check_cam above angled down/3(TipCamSph)
  grab_check_cam above angled down/1(grab ok) -> Mux/2, Grab possible/1
  cam2obj/1 -> FoV/1(spherical coord), grab_check_cam above angled down/1(CamObjSph)
  objPose/1 -> grab_check_cam above angled down/2(ObjPose)
  FoV/1(Obj_visible) -> Visible/1, Mux/1
  Mux/1 -> Score/1(In1)
  Score/1(Out1) -> Points/1
  grab_check_cam above angled down/4(Bonus) -> Score/2(In2)
  Score/2(Out2) -> uncapped/1

== system AariaHIABR2017a/Subsystem2 ==
  GrabPossible : Inport
  GrabInput : Inport  Port=2
  Logical Operator : Logic  AllPortsSameDT=off  OutDataTypeStr=boolean
  Manual Switch : ManualSwitch
  Memory : Memory
  Subsystem1 : Subsystem
  Out : Outport
  wires:
  Subsystem1/1(Out1) -> Out/1
  Logical Operator/1 -> Manual Switch/1
  GrabInput/1 -> Manual Switch/2, Logical Operator/1
  Manual Switch/1 -> Memory/1
  Memory/1 -> Subsystem1/Trigger
  GrabPossible/1 -> Logical Operator/2
